simulink library "sm_rollerV_lib_underc_idlerArm_i2u0l3"  (R2026a)
settings: Solver=VariableStepAuto
undefined symbols (not defined in the file): Fixed, P1, P2, P3, P4, P5, Right, Trac, X, Y, Z
libraries: sm_rollerV_lib_underc_elem x11, sm_lib x11, nesl_utility x7, sm_trackV_lib_belt_underc_elem x4, fl_lib x2, sm_trackV_lib_frame_idlerArm_i2u0l3 x1
(part 1 of 2)
Description:
  | Copyright 2023-2026 The MathWorks, Inc.
settings Model: Creator=smiller  LastModifiedBy=smiller

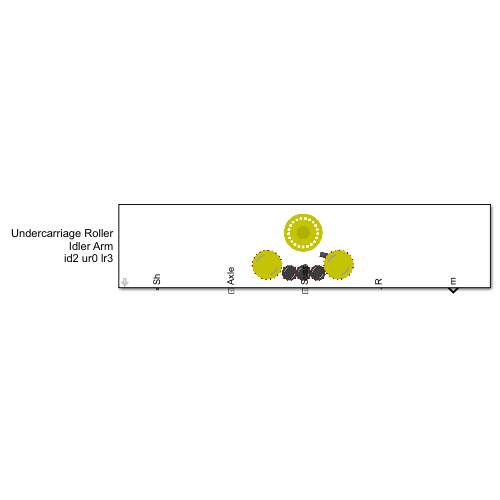
[thumbnail: Simulink's stored preview of the top-level diagram]
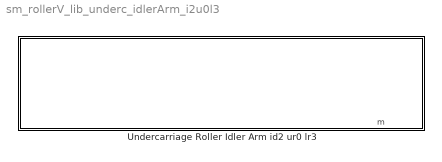
== system sm_rollerV_lib_underc_idlerArm_i2u0l3 ==
  Undercarriage Roller Idler Arm id2 ur0 lr3 : Subsystem  mask(Undercarriage with Roller Ground Contact (Point Cloud)){popup_leftOrRight=Right, sprk_rad_roll=Trac.Sprocket.Roller.rad, sprk_wid_roll=Trac.Sprocket.Roller.wid, sprk_clr=Trac.Sprocket.Roller.clr, sprk_opc=Trac.Sprocket.Roller.opc, sprk_rim_ir=Trac.Sprocket.Rim.rad_inner, sprk_rim_thk=Trac.Sprocket.Rim.thk, sprk_rim_spoke_xc=Trac.Sprocket.Rim.spoke_xc, sprk_rad_pitch=Trac.Sprocket.Spoke.pitch_rad, sprk_spoke_rad=Trac.Sprocket.Spoke.rad, sprk_spoke_len=Trac.Sprocket.Spoke.len, sprk_spoke_num=Trac.Sprocket.nSpokes, idlerR_rad=Trac.IdlerR.rad, idlerF_rad=Trac.IdlerF.rad, idlerR_total_len=Trac.IdlerR.len_total, idlerF_total_len=Trac.IdlerF.len_total, idlerR_avg_rho=Trac.IdlerR.rho_avg, idlerF_avg_rho=Trac.IdlerF.rho_avg, idlerR_clr=Trac.IdlerR.clr, idlerF_clr=Trac.IdlerF.clr, idlerR_opc=Trac.IdlerR.opc, idlerF_opc=Trac.IdlerF.opc, idlerR_contgeo_ptcld=Trac.IdlerR.ground_contact.ptcld.pts, idlerF_contgeo_ptcld=Trac.IdlerF.ground_contact.ptcld.pts, idlerR_contgeo_rad=Trac.IdlerR.ground_contact.ptcld.rad, idlerF_contgeo_rad=Trac.IdlerF.ground_contact.ptcld.rad, idlerR_contgeo_clr=Trac.IdlerR.belt_contact.clr, idlerF_contgeo_clr=Trac.IdlerF.belt_contact.clr, idlerR_contgeo_opc=Trac.IdlerR.belt_contact.opc, idlerF_contgeo_opc=Trac.IdlerF.belt_contact.opc, arm_idlerc=Trac.IdlerArm.Pivot_to_Idler, arm_tens_x=Trac.IdlerArm.Pivot_to_TensionerX, arm_tens_y=Trac.IdlerArm.Pivot_to_TensionerY, arm_wid=Trac.IdlerArm.wid, arm_thk=Trac.IdlerArm.thk, arm_rho=Trac.IdlerArm.rho, arm_clr=Trac.IdlerArm.clr, arm_opc=Trac.IdlerArm.opc, roller_lower_len=Trac.Roller.Lower.len, roller_lower_rad=Trac.Roller.Lower.rad, roller_lower_rho=Trac.Roller.Lower.rho, roller_lower_clr=Trac.Roller.Lower.clr, roller_lower_opc=Trac.Roller.Lower.opc, roller_lower_contgeo_clr=Trac.Roller.Lower.belt_contact.clr, roller_lower_contgeo_opc=Trac.Roller.Lower.belt_contact.opc, roller_lower_contgeo_ptcld=Trac.Roller.Lower.ground_contact.ptcld.pts, roller_lower_contgeo_rad=Trac.Roller.Lower.ground_contact.ptcld.rad, tensioner_cyl_len=Trac.IdlerF.Tensioner.cyl.len, tensioner_cyl_rad=Trac.IdlerF.Tensioner.cyl.rad, tensioner_cyl_rho=Trac.IdlerF.Tensioner.cyl.rho, tensioner_cyl_clr=Trac.IdlerF.Tensioner.cyl.clr, tensioner_cyl_opc=Trac.IdlerF.Tensioner.cyl.opc, tensioner_pist_len=Trac.IdlerF.Tensioner.piston.len, tensioner_pist_rad=Trac.IdlerF.Tensioner.piston.rad, tensioner_pist_rho=Trac.IdlerF.Tensioner.piston.rho, tensioner_pist_clr=Trac.IdlerF.Tensioner.piston.clr, tensioner_pist_opc=Trac.IdlerF.Tensioner.piston.opc, tensioner_br_len=Trac.IdlerF.Tensioner.bracket.len, tensioner_br_width=Trac.IdlerF.Tensioner.bracket.wid, tensioner_br_height=Trac.IdlerF.Tensioner.bracket.height, tensioner_br_thk=Trac.IdlerF.Tensioner.bracket.thk, tensioner_br_rho=Trac.IdlerF.Tensioner.bracket.rho, tensioner_br_clr=Trac.IdlerF.Tensioner.bracket.clr, tensioner_br_opc=Trac.IdlerF.Tensioner.bracket.opc, tensioner_eqpos=Trac.IdlerF.Tensioner.xeq, tensioner_x0=Trac.IdlerF.Tensioner.x0, tensioner_k=Trac.IdlerF.Tensioner.K, tensioner_b=Trac.IdlerF.Tensioner.B, popup_trackFrame=Fixed, roller_lower_x=Trac.Frame.SprkOffLon.Lower, axle_x=Trac.Frame.SprkOffLon.Axle, idlerFix_x=Trac.Frame.SprkOffLon.IdlerR, frame_pivot_x=Trac.Frame.SprkOffLon.PivotFra, tensionC_x=Trac.Frame.SprkOffLon.TensionC, idlerArm_x=Trac.Frame.SprkOffLon.IdlerArm, roller_lower_y=Trac.Frame.SprkOffVer.Lower, axle_y=Trac.Frame.SprkOffVer.Axle, idlerArm_y=Trac.Frame.SprkOffVer.IdlerArm, idlerFix_y=Trac.Frame.SprkOffVer.IdlerR, frame_pivot_y=Trac.Frame.SprkOffVer.PivotFra, tensionC_y=Trac.Frame.SprkOffVer.TensionC, frame_cg_offset=Trac.Frame.TrackFrame.CG, frame_mass=Trac.Frame.TrackFrame.Mass, frame_moi=Trac.Frame.TrackFrame.MOI, frame_poi=Trac.Frame.TrackFrame.POI, frame_roller_cg_offset=Trac.Frame.SprkFrame.CG, frame_roller_mass=Trac.Frame.SprkFrame.Mass, frame_roller_moi=Trac.Frame.SprkFrame.MOI, frame_roller_poi=Trac.Frame.SprkFrame.POI, frame_susp_offset=Trac.Frame.SuspOffset, roller_frame_pivot_range=Trac.Frame.PivotFra.Range, roller_frame_pivot_k=Trac.Frame.PivotFra.LimitK, roller_frame_pivot_b=Trac.Frame.PivotFra.LimitB, roller_frame_pivot_tw=Trac.Frame.PivotFra.LimitTW, sprk_rolling_rad=Trac.Sprocket.ground_contact.rolling_radius, roller_lower_rolling_rad=Trac.Roller.Lower.ground_contact.rolling_radius, idlerF_rolling_rad=Trac.IdlerF.ground_contact.rolling_radius, idlerR_rolling_rad=Trac.IdlerR.ground_contact.rolling_radius, rolling_cyl_len=Trac.Belt.w, accent_vis_lext=1e-3, roller_lower_cyl_clr=Trac.Roller.Lower.clr, roller_lower_cyl_opc=Trac.Roller.Lower.opc, idlerR_rollvervis_clr=Trac.IdlerR.clr, idlerF_rollvervis_clr=Trac.IdlerF.clr, idlerR_rollervis_opc=Trac.IdlerR.opc, idlerF_rollervis_opc=Trac.IdlerF.opc, accMn=0.65, accMx=0.75, acc_clr=[0.8 0.8 0.8], acc_opc=1, popup_sense_roller=Actuator Torque}
      mask prompts: popup_leftOrRight "Left or Right"; sprk_rad_roll "Rolling Radius (m)"; sprk_wid_roll "Roller Width (m)"; sprk_clr "Color [R G B] (0-1)"; sprk_opc "Roller Opacity (0-1)"; sprk_rim_ir "Inner Radius (m)"; sprk_rim_thk "Thickness (m)"; sprk_rim_spoke_xc "Spoke Cross Section [x y] (m)"; sprk_rad_pitch "Pitch Radius (m)"; sprk_spoke_rad "Radius (m)"; sprk_spoke_len "Length (m)"; sprk_spoke_num "Number of Spokes"; arm_idlerc "Offset Pivot to Idler Center (m)"; arm_tens_x "Offset Pivot to Tensioner Long. (m)"; arm_tens_y "Offset Pivot to Tensioner Vert. (m)"; arm_wid "Idler Arm Width (m)"; arm_thk "Idler Arm Thickness (m)"; arm_rho "Idler Arm Density"; arm_clr "Idler Arm Color [R G B] (m) (0-1)"; arm_opc "Opacity (0-1)"; roller_lower_len "Length (m)"; roller_lower_rad "Radius (m)"; roller_lower_rho "Density (kg/m^3)"; roller_lower_clr "Color [R G B] (0-1)"; roller_lower_opc "Opacity (0-1)"; roller_lower_contgeo_clr "Color [R G B] (0-1)"; roller_lower_contgeo_opc "Opacity (0-1)"; roller_lower_contgeo_ptcld "Point Cloud [x y z] (m)"; roller_lower_contgeo_rad "Radius (m)"; tensioner_cyl_len "Length (m)"; tensioner_cyl_rad "Radius (m)"; tensioner_cyl_rho "Density (kg/m^3)"; tensioner_cyl_clr "Color [R G B] (0-1)"; tensioner_cyl_opc "Opacity (0-1)"; tensioner_pist_len "Piston Length (m)"; tensioner_pist_rad "Radius (m)"; tensioner_pist_rho "Density (kg/m^3)"; tensioner_pist_clr "Color [R G B] (0-1)"; tensioner_pist_opc "Opacity (0.1)"; tensioner_br_len "Length (m)"; tensioner_br_width "Width (m)"; tensioner_br_height "Height (m)"; tensioner_br_thk "Bracket Thickness (m)"; tensioner_br_rho "Density (kg/m^3)"; tensioner_br_clr "Color [R G B] (0-1)"; tensioner_br_opc "Opacity (0.1)"; tensioner_eqpos "Equilibrium Position (m)"; tensioner_x0 "Assembly Position (m)"; tensioner_k "Stiffness Coefficient (N/m)"; tensioner_b "Damping Coefficient (N/(m/s))"; popup_trackFrame "Track Frame"; roller_lower_x "Lower Rollers (vector) (m)"; axle_x "Axle (m)"; idlerFix_x "Idler Wheel Fixed (m)"; frame_pivot_x "Frame Pivot (m)"; tensionC_x "Tensioner Cylinder (m)"; idlerArm_x "Idler Arm (m)"; roller_lower_y "Lower Rollers (m)"; axle_y "Axle (m)"; idlerArm_y "Idler Arm (m)"; idlerFix_y "Idler Wheel Fixed (m)"; frame_pivot_y "Frame Pivot (m)"; tensionC_y "Tensioner Cylinder (m)"; frame_cg_offset "CG Offset from Sprocket [x y z] (m)"; frame_mass "Mass (kg)"; frame_moi "Moments of Inertia [Ixx Iyy Izz] (kg*m^2)"; frame_poi "Products of Inertia [Ixx Iyy Izz] (kg*m^2)"; frame_roller_cg_offset "CG Offset from Sprocket [x y z] (m)"; frame_roller_mass "Mass (kg)"; frame_roller_moi "Moments of Inertia [Ixx Iyy Izz] (kg*m^2)"; frame_roller_poi "Products of Inertia [Ixx Iyy Izz] (kg*m^2)"; frame_susp_offset "Suspension Offset from Sprocket [x y z] (m)"; roller_frame_pivot_range "Range (deg)"; roller_frame_pivot_k "Stop stiffness (N*m/deg)"; roller_frame_pivot_b "Stop damping (N*m/(deg*sec)"; roller_frame_pivot_tw "Stop transition width (deg)"; sprk_rolling_rad "Sprocket Rolling Radius (m)"; roller_lower_rolling_rad "Lower Roller Rolling Radius (m)"; idlerF_rolling_rad "Front Idler Rolling Radius (m)"; idlerR_rolling_rad "Rear Idler Rolling Radius (m)"; rolling_cyl_len "Cylinder Length (m)"; accent_vis_lext "Length Extensions (m)"; roller_lower_cyl_clr "Cylinder Color [R G B] (0-1)"; roller_lower_cyl_opc "Cylinder Opacity (0-1)"; accMn "Accent Min Radius (0-1)"; accMx "Accent Max Radius (0-1)"; acc_clr "Accent Color [R G B] (0-1)"; acc_opc "Accent Opacity (0-1)"; popup_sense_roller "Roller"
      mask help: Models sprocket, rollers, fixed idler. and idler on an arm with a tensioner. Components have point cloud contact geometry to enable undercarriage to roll along uneven ground. The sprocket has a 1D rotational mechanical interface to the drivetrain.
      mask TypeOptions popup_leftOrRight: Frame/popup_leftOrRight
      mask TypeOptions sprk_rad_roll: Rollers/sprk_rad_roll
      mask TypeOptions sprk_wid_roll: Rollers/sprk_wid_roll
      mask TypeOptions sprk_clr: Rollers/sprk_clr
      mask TypeOptions sprk_opc: Rollers/sprk_opc
      mask TypeOptions sprk_rim_ir: Rollers/sprk_rim_ir
      mask TypeOptions sprk_rim_thk: Rollers/sprk_rim_thk
      mask TypeOptions sprk_rim_spoke_xc: Rollers/sprk_rim_spoke_xc
      mask TypeOptions sprk_rad_pitch: Rollers/sprk_rad_pitch
      mask TypeOptions sprk_spoke_rad: Rollers/sprk_spoke_rad
      mask TypeOptions sprk_spoke_len: Rollers/sprk_spoke_len
      mask TypeOptions sprk_spoke_num: Rollers/sprk_spoke_num
      mask TypeOptions idlerR_rad: Rollers/idlerR_rad
      mask TypeOptions idlerF_rad: Rollers/idlerF_rad
      mask TypeOptions idlerR_total_len: Rollers/idlerR_total_len
      mask TypeOptions idlerF_total_len: Rollers/idlerF_total_len
      mask TypeOptions idlerR_avg_rho: Rollers/idlerR_avg_rho
      mask TypeOptions idlerF_avg_rho: Rollers/idlerF_avg_rho
      mask TypeOptions idlerR_clr: Rollers/idlerR_clr
      mask TypeOptions idlerF_clr: Rollers/idlerF_clr
      mask TypeOptions idlerR_opc: Rollers/idlerR_opc
      mask TypeOptions idlerF_opc: Rollers/idlerF_opc
      mask TypeOptions idlerR_contgeo_ptcld: Rollers/idlerR_contgeo_ptcld
      mask TypeOptions idlerF_contgeo_ptcld: Rollers/idlerF_contgeo_ptcld
      mask TypeOptions idlerR_contgeo_rad: Rollers/idlerR_contgeo_rad
      mask TypeOptions idlerF_contgeo_rad: Rollers/idlerF_contgeo_rad
      mask TypeOptions idlerR_contgeo_clr: Rollers/idlerR_contgeo_clr
      mask TypeOptions idlerF_contgeo_clr: Rollers/idlerF_contgeo_clr
      mask TypeOptions idlerR_contgeo_opc: Rollers/idlerR_contgeo_opc
      mask TypeOptions idlerF_contgeo_opc: Rollers/idlerF_contgeo_opc
      mask TypeOptions arm_idlerc: Rollers/arm_idlerc
      mask TypeOptions arm_tens_x: Rollers/arm_tens_x
      mask TypeOptions arm_tens_y: Rollers/arm_tens_y
      mask TypeOptions arm_wid: Rollers/arm_wid
      mask TypeOptions arm_thk: Rollers/arm_thk
      mask TypeOptions arm_rho: Rollers/arm_rho
      mask TypeOptions arm_clr: Rollers/arm_clr
      mask TypeOptions arm_opc: Rollers/arm_opc
      mask TypeOptions roller_lower_len: Rollers/roller_lower_len
      mask TypeOptions roller_lower_rad: Rollers/roller_lower_rad
      mask TypeOptions roller_lower_rho: Rollers/roller_lower_rho
      mask TypeOptions roller_lower_clr: Rollers/roller_lower_clr
      mask TypeOptions roller_lower_opc: Rollers/roller_lower_opc
      mask TypeOptions roller_lower_contgeo_clr: Rollers/roller_lower_contgeo_clr
      mask TypeOptions roller_lower_contgeo_opc: Rollers/roller_lower_contgeo_opc
      mask TypeOptions roller_lower_contgeo_ptcld: Rollers/roller_lower_contgeo_ptcld
      mask TypeOptions roller_lower_contgeo_rad: Rollers/roller_lower_contgeo_rad
      mask TypeOptions tensioner_cyl_len: Rollers/tensioner_cyl_len
      mask TypeOptions tensioner_cyl_rad: Rollers/tensioner_cyl_rad
      mask TypeOptions tensioner_cyl_rho: Rollers/tensioner_cyl_rho
      mask TypeOptions tensioner_cyl_clr: Rollers/tensioner_cyl_clr
      mask TypeOptions tensioner_cyl_opc: Rollers/tensioner_cyl_opc
      mask TypeOptions tensioner_pist_len: Rollers/pist_len
      mask TypeOptions tensioner_pist_rad: Rollers/tensioner_pist_rad
      mask TypeOptions tensioner_pist_rho: Rollers/tensioner_pist_rho
      mask TypeOptions tensioner_pist_clr: Rollers/tensioner_pist_clr
      mask TypeOptions tensioner_pist_opc: Rollers/tensioner_pist_opc
      mask TypeOptions tensioner_br_len: Rollers/brk_len
      mask TypeOptions tensioner_br_width: Rollers/tensioner_br_width
      mask TypeOptions tensioner_br_height: Rollers/tensioner_br_height
      mask TypeOptions tensioner_br_thk: Rollers/brk_thk
      mask TypeOptions tensioner_br_rho: Rollers/tensioner_br_rho
      mask TypeOptions tensioner_br_clr: Rollers/tensioner_br_clr
      mask TypeOptions tensioner_br_opc: Rollers/tensioner_br_opc
      mask TypeOptions tensioner_eqpos: Rollers/tensioner_eqpos
      mask TypeOptions tensioner_x0: Rollers/tensioner_x0
      mask TypeOptions tensioner_k: Rollers/tensioner_k
      mask TypeOptions tensioner_b: Rollers/tensioner_b
      mask TypeOptions popup_trackFrame: Frame/popup_trackFrame
      mask TypeOptions roller_lower_x: Frame/roller_lower_x
      mask TypeOptions axle_x: Frame/axle_x
      mask TypeOptions idlerFix_x: Frame/idlerFix_x
      mask TypeOptions frame_pivot_x: Frame/frame_pivot_x
      mask TypeOptions tensionC_x: Frame/tensionC_x
      mask TypeOptions idlerArm_x: Frame/idlerArm_x
      mask TypeOptions roller_lower_y: Frame/roller_lower_y
      mask TypeOptions axle_y: Frame/axle_y
      mask TypeOptions idlerArm_y: Frame/idlerArm_y
      mask TypeOptions idlerFix_y: Frame/idlerFix_y
      mask TypeOptions frame_pivot_y: Frame/frame_pivot_y
      mask TypeOptions tensionC_y: Frame/tensionC_y
      mask TypeOptions frame_cg_offset: Frame/frame_cg_offset
      mask TypeOptions frame_mass: Frame/frame_mass
      mask TypeOptions frame_moi: Frame/frame_moi
      mask TypeOptions frame_poi: Frame/frame_poi
      mask TypeOptions frame_roller_cg_offset: Frame/frame_roller_cg_offset
      mask TypeOptions frame_roller_mass: Frame/frame_roller_mass
      mask TypeOptions frame_roller_moi: Frame/frame_roller_moi
      mask TypeOptions frame_roller_poi: Frame/frame_roller_poi
      mask TypeOptions frame_susp_offset: Frame/frame_susp_offset
      mask TypeOptions roller_frame_pivot_range: Frame/roller_frame_pivot_range
      mask TypeOptions roller_frame_pivot_k: Frame/roller_frame_pivot_k
      mask TypeOptions roller_frame_pivot_b: Frame/roller_frame_pivot_b
      mask TypeOptions roller_frame_pivot_tw: Frame/roller_frame_pivot_tw
      mask TypeOptions sprk_rolling_rad: Rollers/sprk_rolling_rad
      mask TypeOptions roller_lower_rolling_rad: Rollers/roller_lower_rolling_rad
      mask TypeOptions idlerF_rolling_rad: Rollers/idlerF_rolling_rad
      mask TypeOptions idlerR_rolling_rad: Rollers/idlerR_rolling_rad
      mask TypeOptions rolling_cyl_len: Rollers/cyl_len
      mask TypeOptions accent_vis_lext: Rollers/lext
      mask TypeOptions roller_lower_cyl_clr: Rollers/roller_lower_cyl_clr
      mask TypeOptions roller_lower_cyl_opc: Rollers/roller_lower_cyl_opc
      mask TypeOptions idlerR_rollvervis_clr: Rollers/idlerR_rollvervis_clr
      mask TypeOptions idlerF_rollvervis_clr: Rollers/idlerF_rollvervis_clr
      mask TypeOptions idlerR_rollervis_opc: Rollers/idlerR_rollervis_opc
      mask TypeOptions idlerF_rollervis_opc: Rollers/idlerF_rollervis_opc
      mask TypeOptions accMn: Rollers/accMn
      mask TypeOptions accMx: Rollers/accMx
      mask TypeOptions acc_clr: Rollers/acc_clr
      mask TypeOptions acc_opc: Rollers/acc_opc
      mask TypeOptions popup_sense_roller: Rollers/popup_sense_roller
      mask DialogControl cont_sprocket Prompt: Sprocket
      mask DialogControl cont_sprk_roller Prompt: Roller
      mask DialogControl cont_sprk_rim Prompt: Rim
      mask DialogControl cont_sprk_spoke Prompt: Spoke
      mask DialogControl cont_idler Prompt: Idler
      mask DialogControl cont_idler_roller Prompt: Roller
      mask DialogControl text_rear Prompt: Rear
      mask DialogControl text_front Prompt: Front
      mask DialogControl text_rad Prompt: Radius (m)
      mask DialogControl text_len Prompt: Total Length (m)
      mask DialogControl text_rho Prompt: Density (kg/m^3)
      mask DialogControl text_idler_clr Prompt: Color [R G B] (0-1)
      mask DialogControl text_idler_opc Prompt: Opacity (0-1)
      mask DialogControl cont_idler_contact_geo Prompt: Contact Geometry
      mask DialogControl text_idler_contgeo_ptcld Prompt: Point Cloud [x y z] (m)
      mask DialogControl text_idler_contgeo_rad Prompt: Radius (m)
      mask DialogControl text_contgeo_clr_copy Prompt: Color [R G B] (0-1)
      mask DialogControl text_contgeo_opc Prompt: Opacity (0-1)
      mask DialogControl cont_idler_arm Prompt: Idler Arm
      mask DialogControl cont_rollers Prompt: Rollers
      mask DialogControl cont_rollers_lower Prompt: Lower
      mask DialogControl cont_rollers_lower_contact_geo Prompt: Contact Geometry
      mask DialogControl cont_tensioner Prompt: Tensioner
      mask DialogControl cont_tensioner_cyl Prompt: Cylinder
      mask DialogControl cont_tensioner_pist Prompt: Piston
      mask DialogControl cont_tensioner_brkt Prompt: Bracket
      mask DialogControl cont_tensioner_assembly Prompt: Assembly
      mask DialogControl cont_frame Prompt: Frame
      mask DialogControl cont_offset_x Prompt: Longitudinal Offsets from Sprocket
      mask DialogControl cont_offset_y Prompt: Vertical Offsets
      mask DialogControl cont_mass Prompt: Mass and Inertia
      mask DialogControl cont_frame_sprk Prompt: Sprocket Frame
      mask DialogControl cont_frame_roller Prompt: Roller Frame
      mask DialogControl cont_susp Prompt: Suspension Offsets
      mask DialogControl cont_frame_pivot Prompt: Frame Pivot
      mask DialogControl cont_rolling Prompt: Rolling
      mask DialogControl cont_constraints_length Prompt: Constraints and Length
      mask DialogControl cont_rollervis_roller Prompt: Roller Visual: Roller
      mask DialogControl cont_rollervis_idler Prompt: Roller Visual: Idler
      mask DialogControl text_idler_rollervis_rear Prompt: Rear
      mask DialogControl text_idler_rollervis_front Prompt: Front
      mask DialogControl text_idler_rollervis_clr Prompt: Color [R G B] (0-1)
      mask DialogControl text_idler_rollervis_opc Prompt: Opacity (0-1)
      mask DialogControl cont_accentvis Prompt: Accent Visual
      mask DialogControl cont_sensing Prompt: Sensing
      mask Display: image('sm_roller_ptcld_rollers_idlerarm_i2u0l3_IMAGE.png')

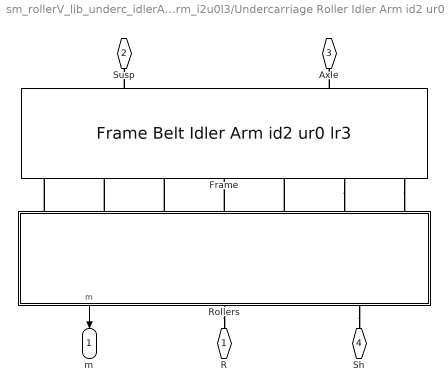
== system sm_rollerV_lib_underc_idlerArm_i2u0l3/Undercarriage Roller Idler Arm id2 ur0 lr3 ==
  Frame : sm_trackV_lib_frame_idlerArm_i2u0l3/Frame Belt Idler Arm id2 ur0 lr3  popup_leftOrRight=Right  popup_trackFrame=Fixed  roller_lower_x=roller_lower_x  idlerArm_x=idlerArm_x  idlerFix_x=idlerFix_x  tensionC_x=tensionC_x  frame_pivot_x=frame_pivot_x  axle_x=axle_x  roller_lower_y=roller_lower_y  idlerArm_y=idlerArm_y  idlerFix_y=idlerFix_y  tensionC_y=tensionC_y  frame_pivot_y=frame_pivot_y  axle_y=axle_y  frame_roller_cg_offset=frame_roller_cg_offset  frame_roller_mass=frame_roller_mass  frame_roller_moi=frame_roller_moi  frame_roller_poi=frame_roller_poi  frame_cg_offset=frame_cg_offset  frame_mass=frame_mass  frame_moi=frame_moi  frame_poi=frame_poi  frame_susp_offset=frame_susp_offset  roller_frame_pivot_range=roller_frame_pivot_range  roller_frame_pivot_k=roller_frame_pivot_k  roller_frame_pivot_b=roller_frame_pivot_b  roller_frame_pivot_tw=roller_frame_pivot_tw
  Rollers : Subsystem  mask(Rollers for Integration with Track Model){sprk_wid_roll=sprk_wid_roll, sprk_rad_roll=sprk_rad_roll, sprk_clr=sprk_clr, sprk_opc=sprk_opc, sprk_rim_ir=sprk_rim_ir, sprk_rim_spoke_xc=sprk_rim_spoke_xc, sprk_rim_thk=sprk_rim_thk, sprk_rad_pitch=sprk_rad_pitch, sprk_spoke_rad=sprk_spoke_rad, sprk_spoke_len=sprk_spoke_len, sprk_spoke_num=sprk_spoke_num, idlerR_rad=idlerR_rad, idlerF_rad=idlerF_rad, idlerR_total_len=idlerR_total_len, idlerF_total_len=idlerF_total_len, idlerR_avg_rho=idlerR_avg_rho, idlerF_avg_rho=idlerF_avg_rho, idlerR_clr=idlerR_clr, idlerF_clr=idlerF_clr, idlerR_opc=idlerR_opc, idlerF_opc=idlerF_opc, idlerR_contgeo_ptcld=idlerR_contgeo_ptcld, idlerF_contgeo_ptcld=idlerF_contgeo_ptcld, idlerR_contgeo_rad=idlerR_contgeo_rad, idlerF_contgeo_rad=idlerF_contgeo_rad, idlerR_contgeo_clr=idlerR_contgeo_clr, idlerF_contgeo_clr=idlerF_contgeo_clr, idlerR_contgeo_opc=idlerR_contgeo_opc, idlerF_contgeo_opc=idlerF_contgeo_opc, arm_idlerc=arm_idlerc, arm_tens_x=arm_tens_x, arm_tens_y=arm_tens_y, arm_wid=arm_wid, arm_thk=arm_thk, arm_rho=arm_rho, arm_clr=arm_clr, arm_opc=arm_opc, roller_lower_len=roller_lower_len, roller_lower_rad=roller_lower_rad, roller_lower_rho=roller_lower_rho, roller_lower_clr=roller_lower_clr, roller_lower_opc=roller_lower_opc, roller_lower_contgeo_ptcld=roller_lower_contgeo_ptcld, roller_lower_contgeo_rad=roller_lower_contgeo_rad, roller_lower_contgeo_clr=roller_lower_contgeo_clr, roller_lower_contgeo_opc=roller_lower_contgeo_opc, tensioner_cyl_rad=tensioner_cyl_rad, tensioner_cyl_len=tensioner_cyl_len, tensioner_cyl_rho=tensioner_cyl_rho, tensioner_cyl_clr=tensioner_cyl_clr, tensioner_cyl_opc=tensioner_cyl_opc, tensioner_pist_rad=tensioner_pist_rad, pist_len=tensioner_pist_len, tensioner_pist_rho=tensioner_pist_rho, tensioner_pist_clr=tensioner_pist_clr, tensioner_pist_opc=tensioner_pist_opc, brk_len=tensioner_br_len, tensioner_br_width=tensioner_br_width, tensioner_br_height=tensioner_br_height, brk_thk=tensioner_br_thk, tensioner_br_rho=tensioner_br_rho, tensioner_br_clr=tensioner_br_clr, tensioner_br_opc=tensioner_br_opc, tensioner_eqpos=tensioner_eqpos, tensioner_x0=tensioner_x0, tensioner_b=tensioner_b, tensioner_k=tensioner_k, sprk_rolling_rad=sprk_rolling_rad, roller_lower_rolling_rad=roller_lower_rolling_rad, idlerF_rolling_rad=idlerF_rolling_rad, idlerR_rolling_rad=idlerR_rolling_rad, cyl_len=rolling_cyl_len, roller_lower_cyl_clr=roller_lower_cyl_clr, roller_lower_cyl_opc=roller_lower_cyl_opc, idlerR_rollvervis_clr=idlerR_rollvervis_clr, idlerF_rollvervis_clr=idlerF_rollvervis_clr, idlerR_rollervis_opc=idlerR_rollervis_opc, idlerF_rollervis_opc=idlerF_rollervis_opc, accMn=accMn, accMx=accMx, acc_clr=acc_clr, acc_opc=acc_opc, lext=accent_vis_lext, popup_sense_roller=Actuator Torque}
      mask prompts: sprk_wid_roll "Roller Width (m)"; sprk_rad_roll "Rolling Radius (m)"; sprk_clr "Roller Color [R G B] (0-1)"; sprk_opc "Roller Opacity (0-1)"; sprk_rim_ir "Inner Radius (m)"; sprk_rim_spoke_xc "Spoke Cross Section [x y] (m)"; sprk_rim_thk "Thickness (m)"; sprk_rad_pitch "Pitch Radius (m)"; sprk_spoke_rad "Radius (m)"; sprk_spoke_len "Length (m)"; sprk_spoke_num "Number of Spokes"; arm_idlerc "Offset Pivot to Idler Center (m)"; arm_tens_x "Offset Pivot to Tensioner Long.  (m)"; arm_tens_y "Offset Pivot to Tensioner Vert.  (m)"; arm_wid "Idler Arm Width (m)"; arm_thk "Idler Arm Thickness (m)"; arm_rho "Idler Arm Density (kg/m^3)"; arm_clr "Idler Arm Color [R G B] (0-1)"; arm_opc "Idler Arm Opacity (0-1)"; roller_lower_len "Length (m)"; roller_lower_rad "Radius (m)"; roller_lower_rho "Density (kg/m^3)"; roller_lower_clr "Color [R G B] (0-1)"; roller_lower_opc "Opacity (0-1)"; roller_lower_contgeo_ptcld "Point Cloud [x y z] (m)"; roller_lower_contgeo_rad "Radius (m)"; roller_lower_contgeo_clr "Color [R G B] (0-1)"; roller_lower_contgeo_opc "Opacity (0-1)"; tensioner_cyl_rad "Radius (m)"; tensioner_cyl_len "Length (m)"; tensioner_cyl_rho "Density (kg/m^3)"; tensioner_cyl_clr "Color [R G B] (0-1)"; tensioner_cyl_opc "Opacity (0-1)"; tensioner_pist_rad "Radius (m)"; pist_len "Piston Length (m)"; tensioner_pist_rho "Density (kg/m^3)"; tensioner_pist_clr "Color [R G B] (0-1)"; tensioner_pist_opc "Opacity (0.1)"; brk_len "Bracket Length (m)"; tensioner_br_width "Width (m)"; tensioner_br_height "Height (m)"; brk_thk "Bracket Thickness (m)"; tensioner_br_rho "Density (kg/m^3)"; tensioner_br_clr "Color [R G B] (0-1)"; tensioner_br_opc "Opacity (0.1)"; tensioner_eqpos "Equilibrium Position (m)"; tensioner_x0 "Assembly Position (m)"; tensioner_b "Damping Coefficient (N/(m/s))"; tensioner_k "Stiffness Coefficient (N/m)"; sprk_rolling_rad "Sprocket Rolling Radius (m)"; roller_lower_rolling_rad "Lower Roller Rolling Radius (m)"; idlerF_rolling_rad "Front Idler Rolling Radius (m)"; idlerR_rolling_rad "Rear Idler Rolling Radius (m)"; cyl_len "Cylinder Length (m)"; roller_lower_cyl_clr "Cylinder Color [R G B] (0-1)"; roller_lower_cyl_opc "Cylinder Opacity (0-1)"; accMn "Accent Min Radius (0-1)"; accMx "Accent Max Radius (0-1)"; acc_clr "Accent Color [R G B] (0-1)"; acc_opc "Accent Opacity (0-1)"; lext "Length Extensions (m)"; popup_sense_roller "Roller"
      mask help: Models sprocket, rollers, and idler with tensioner. Components have contact geometry for integration with a segmented track model. The sprocket has a 1D rotational mechanical interface to the drivetrain.
      mask init:
      | % Sensing a constraint force can be computationally expensive
      | % Use popup to turn it off if quantity is not needed
      | 
      | bh = gcb;
      | if(strcmp(get_param(bh,'popup_sense_roller'),'Constraint Force'))
      |     SCF = 'on'; STF = 'off';
      |     connectedPort = "fc_out";
      |     senseConstraintTorque = "on";
      |     senseTorqueForce = "off";
      | 
      | else
      |     SCF = 'off'; STF = 'on';
      |     connectedPort = "t_out";
      |     senseConstraintTorque = "off";
      |     senseTorqueForce = "on";
      | end
      | 
      | f = Simulink.FindOptions('RegExp',true,'SearchDepth',1);
      | bh_rv = Simulink.findBlocks(gcb,'Name','Revolute Lower #*',f);
      | bh_ps = Simulink.findBlocks(bh,'Name','PS-SL Lower #*',f);
      | [~, indrv] = sort(getfullname(bh_rv));
      | [~, indps] = sort(getfullname(bh_ps));
      | bh_rv = bh_rv(indrv);
      | bh_ps = bh_ps(indps);
      | 
      | bh_rvidf = get_param([bh '/Revolute Idler F'],'Handle');
      | bh_rvidr = get_param([bh '/Revolute Idler R'],'Handle');
      | 
      | bh_psidf = get_param([bh '/PS-SL IdlerF'],'Handle');
      | bh_psidr = get_param([bh '/PS-SL IdlerR'],'Handle');
      | 
      | bh_rv = [bh_rv; bh_rvidr; bh_rvidf];
      | bh_ps = [bh_ps; bh_psidr; bh_psidf];
      | 
      | for i = 1:length(bh_rv)
      |     port_rv = get_param(bh_rv(i),'PortHandles');
      |     port_ps = get_param(bh_ps(i),'PortHandles');
      |     line_rv = get_param(bh_rv(i),'LineHandles');
      |     delete_line(line_rv.RConn(2))
      |     set_param(bh_rv(i),'SenseConstraintForce',SCF,'SenseTorqueForce',STF);
      |     simscape.addConnection(bh_rv(i), connectedPort, bh_ps(i),'input');
      | end
      mask TypeOptions sprk_wid_roll: Sprocket/sprk_wid_roll
      mask TypeOptions sprk_rad_roll: Sprocket/sprk_rad_roll
      mask TypeOptions sprk_clr: Sprocket/sprk_clr | Sprocket/sprk_spoke_clr
      mask TypeOptions sprk_opc: Sprocket/sprk_opc | Sprocket/sprk_spoke_opc
      mask TypeOptions sprk_rim_ir: Sprocket/rim_ir
      mask TypeOptions sprk_rim_spoke_xc: Sprocket/rim_spoke_xc
      mask TypeOptions sprk_rim_thk: Sprocket/rim_thk
      mask TypeOptions sprk_rad_pitch: Sprocket/sprk_rad_pitch
      mask TypeOptions sprk_spoke_rad: Sprocket/sprk_spoke_rad
      mask TypeOptions sprk_spoke_len: Sprocket/sprk_spoke_len
      mask TypeOptions sprk_spoke_num: Sprocket/sprk_spoke_num
      mask TypeOptions idlerR_rad: IdlerR/roller_lower_rad
      mask TypeOptions idlerF_rad: IdlerF/roller_lower_rad
      mask TypeOptions idlerR_total_len: IdlerR/roller_lower_len
      mask TypeOptions idlerF_total_len: IdlerF/roller_lower_len
      mask TypeOptions idlerR_avg_rho: IdlerR/roller_lower_rho
      mask TypeOptions idlerF_avg_rho: IdlerF/roller_lower_rho
      mask TypeOptions idlerR_clr: IdlerR/roller_lower_clr
      mask TypeOptions idlerF_clr: IdlerF/roller_lower_clr
      mask TypeOptions idlerR_opc: IdlerR/roller_lower_opc
      mask TypeOptions idlerF_opc: IdlerF/roller_lower_opc
      mask TypeOptions idlerR_contgeo_ptcld: IdlerR/roller_lower_contgeo_ptcld
      mask TypeOptions idlerF_contgeo_ptcld: IdlerF/roller_lower_contgeo_ptcld
      mask TypeOptions idlerR_contgeo_rad: IdlerR/roller_lower_contgeo_rad
      mask TypeOptions idlerF_contgeo_rad: IdlerF/roller_lower_contgeo_rad
      mask TypeOptions idlerR_contgeo_clr: IdlerR/roller_lower_contgeo_clr
      mask TypeOptions idlerF_contgeo_clr: IdlerF/roller_lower_contgeo_clr
      mask TypeOptions idlerR_contgeo_opc: IdlerR/roller_lower_contgeo_opc
      mask TypeOptions idlerF_contgeo_opc: IdlerF/roller_lower_contgeo_opc
      mask TypeOptions arm_idlerc: Arm/arm_idlerc
      mask TypeOptions arm_tens_x: Arm/arm_tens_x
      mask TypeOptions arm_tens_y: Arm/arm_tens_y
      mask TypeOptions arm_wid: Arm/arm_wid
      mask TypeOptions arm_thk: Arm/arm_thk
      mask TypeOptions arm_rho: Arm/arm_rho
      mask TypeOptions arm_clr: Arm/arm_clr
      mask TypeOptions arm_opc: Arm/arm_opc
      mask TypeOptions roller_lower_len:
      | Roller
      | Lower 1/roller_lower_len | Roller
      | Lower 2/roller_lower_len | Roller
      | Lower 3/roller_lower_len
      mask TypeOptions roller_lower_rad:
      | Roller
      | Lower 1/roller_lower_rad | Roller
      | Lower 2/roller_lower_rad | Roller
      | Lower 3/roller_lower_rad
      mask TypeOptions roller_lower_rho:
      | Roller
      | Lower 1/roller_lower_rho | Roller
      | Lower 2/roller_lower_rho | Roller
      | Lower 3/roller_lower_rho
      mask TypeOptions roller_lower_clr:
      | Roller
      | Lower 1/roller_lower_clr | Roller
      | Lower 2/roller_lower_clr | Roller
      | Lower 3/roller_lower_clr
      mask TypeOptions roller_lower_opc:
      | Roller
      | Lower 1/roller_lower_opc | Roller
      | Lower 2/roller_lower_opc | Roller
      | Lower 3/roller_lower_opc
      mask TypeOptions roller_lower_contgeo_ptcld:
      | Roller
      | Lower 1/roller_lower_contgeo_ptcld | Roller
      | Lower 2/roller_lower_contgeo_ptcld | Roller
      | Lower 3/roller_lower_contgeo_ptcld
      mask TypeOptions roller_lower_contgeo_rad:
      | Roller
      | Lower 1/roller_lower_contgeo_rad | Roller
      | Lower 2/roller_lower_contgeo_rad | Roller
      | Lower 3/roller_lower_contgeo_rad
      mask TypeOptions roller_lower_contgeo_clr:
      | Roller
      | Lower 1/roller_lower_contgeo_clr | Roller
      | Lower 2/roller_lower_contgeo_clr | Roller
      | Lower 3/roller_lower_contgeo_clr | Roller
      | Lower 4/roller_lower_contgeo_clr
      mask TypeOptions roller_lower_contgeo_opc:
      | Roller
      | Lower 1/roller_lower_contgeo_opc | Roller
      | Lower 2/roller_lower_contgeo_opc | Roller
      | Lower 3/roller_lower_contgeo_opc | Roller
      | Lower 4/roller_lower_contgeo_opc
      mask TypeOptions tensioner_cyl_rad:
      | Tensioner
      | Cylinder/cyl_rad
      mask TypeOptions tensioner_cyl_len:
      | Tensioner
      | Cylinder/cyl_len
      mask TypeOptions tensioner_cyl_rho:
      | Tensioner
      | Cylinder/cyl_rho
      mask TypeOptions tensioner_cyl_clr:
      | Tensioner
      | Cylinder/cyl_clr
      mask TypeOptions tensioner_cyl_opc:
      | Tensioner
      | Cylinder/cyl_opc
      mask TypeOptions tensioner_pist_rad:
      | Tensioner
      | Piston/pist_rad
      mask TypeOptions pist_len:
      | Tensioner
      | Cylinder/pist_len | Tensioner
      | Piston/pist_len
      mask TypeOptions tensioner_pist_rho:
      | Tensioner
      | Piston/pist_rho
      mask TypeOptions tensioner_pist_clr:
      | Tensioner
      | Piston/pist_clr
      mask TypeOptions tensioner_pist_opc:
      | Tensioner
      | Piston/pist_opc
      mask TypeOptions brk_len:
      | Tensioner
      | Cylinder/brk_len | Tensioner
      | Piston/br_length
      mask TypeOptions tensioner_br_width:
      | Tensioner
      | Piston/br_width
      mask TypeOptions tensioner_br_height:
      | Tensioner
      | Piston/br_height
      mask TypeOptions brk_thk:
      | Tensioner
      | Cylinder/brk_thk | Tensioner
      | Piston/br_thk
      mask TypeOptions tensioner_br_rho:
      | Tensioner
      | Piston/br_rho
      mask TypeOptions tensioner_br_clr:
      | Tensioner
      | Piston/br_clr
      mask TypeOptions tensioner_br_opc:
      | Tensioner
      | Piston/br_opc
      mask TypeOptions tensioner_eqpos:
      | Prismatic
      | Tensioner/EquilibriumPosition
      mask TypeOptions tensioner_x0:
      | Prismatic
      | Tensioner/PositionTargetValue
      mask TypeOptions tensioner_b:
      | Prismatic
      | Tensioner/DampingCoefficient
      mask TypeOptions tensioner_k:
      | Prismatic
      | Tensioner/SpringStiffness
      mask TypeOptions sprk_rolling_rad:
      | Constrain
      | Rollers
      | Idlers/sprk_rolling_rad
      mask TypeOptions roller_lower_rolling_rad:
      | Constrain
      | Rollers
      | Idlers/roller_lower_rolling_rad | Roller
      | Lower 1/cyl_rad | Roller
      | Lower 2/cyl_rad | Roller
      | Lower 3/cyl_rad
      mask TypeOptions idlerF_rolling_rad:
      | Constrain
      | Rollers
      | Idlers/idlerF_rolling_rad | IdlerF/cyl_rad
      mask TypeOptions idlerR_rolling_rad:
      | Constrain
      | Rollers
      | Idlers/idlerR_rolling_rad | IdlerR/cyl_rad
      mask TypeOptions cyl_len:
      | IdlerF/cyl_len | IdlerR/cyl_len | Roller
      | Lower 1/cyl_len | Roller
      | Lower 2/cyl_len | Roller
      | Lower 3/cyl_len
      mask TypeOptions roller_lower_cyl_clr:
      | Roller
      | Lower 1/cyl_clr | Roller
      | Lower 2/cyl_clr | Roller
      | Lower 3/cyl_clr
      mask TypeOptions roller_lower_cyl_opc:
      | Roller
      | Lower 1/cyl_opc | Roller
      | Lower 2/cyl_opc | Roller
      | Lower 3/cyl_opc
      mask TypeOptions idlerR_rollvervis_clr: IdlerR/cyl_clr
      mask TypeOptions idlerF_rollvervis_clr: IdlerF/cyl_clr
      mask TypeOptions idlerR_rollervis_opc: IdlerR/cyl_opc
      mask TypeOptions idlerF_rollervis_opc: IdlerF/cyl_opc
      mask TypeOptions accMn:
      | IdlerF/accMn | IdlerR/accMn | Roller
      | Lower 1/accMn | Roller
      | Lower 2/accMn | Roller
      | Lower 3/accMn
      mask TypeOptions accMx:
      | IdlerF/accMx | IdlerR/accMx | Roller
      | Lower 1/accMx | Roller
      | Lower 2/accMx | Roller
      | Lower 3/accMx
      mask TypeOptions acc_clr:
      | IdlerF/acc_clr | IdlerR/acc_clr | Roller
      | Lower 1/acc_clr | Roller
      | Lower 2/acc_clr | Roller
      | Lower 3/acc_clr
      mask TypeOptions acc_opc:
      | IdlerF/acc_opc | IdlerR/acc_opc | Roller
      | Lower 1/acc_opc | Roller
      | Lower 2/acc_opc | Roller
      | Lower 3/acc_opc
      mask TypeOptions lext:
      | IdlerF/lext | IdlerR/lext | Roller
      | Lower 1/lext | Roller
      | Lower 2/lext | Roller
      | Lower 3/lext
      mask TypeOptions popup_sense_roller: Constraint Force | Actuator Torque
      mask DialogControl cont_sprk Prompt: Sprocket
      mask DialogControl sprk_roller Prompt: Roller
      mask DialogControl cont_rim Prompt: Rim
      mask DialogControl sprk_spoke Prompt: Spoke
      mask DialogControl cont_idler Prompt: Idler
      mask DialogControl cont_idler_roller Prompt: Roller
      mask DialogControl text_idler_rear Prompt: Rear
      mask DialogControl text_idler_front Prompt: Front
      mask DialogControl text_radius Prompt: Radius (m)
      mask DialogControl text_len Prompt: Total Length(m)
      mask DialogControl text_rho Prompt: Average Density (kg/m^3)
      mask DialogControl text_idler_clr Prompt: Color [R G B] (0-1)
      mask DialogControl text_idler_opc Prompt: Opacity (0-1)
      mask DialogControl cont_idler_contact_geo Prompt: Contact Geometry
      mask DialogControl text_idler_contgeo_ptcld Prompt: Point Cloud [x y z] (m)
      mask DialogControl text_idler_contgeo_rad Prompt: Radius (m)
      mask DialogControl text_idler_contgeo_clr Prompt: Color [R G B] (0-1)
      mask DialogControl text_idler_contgeo_opc Prompt: Opacity (0-1)
      mask DialogControl cont_idlerArm Prompt: Idler Arm
      mask DialogControl cont_rollers Prompt: Rollers
      mask DialogControl cont_lower Prompt: Lower
      mask DialogControl cont_lower_contact_geo Prompt: Contact Geometry
      mask DialogControl cont_tensioner Prompt: Tensioner
      mask DialogControl cont_tensioner_cyl Prompt: Cylinder
      mask DialogControl cont_tensioner_pist Prompt: Piston
      mask DialogControl cont_tensioner_brkt Prompt: Bracket
      mask DialogControl cont_tensioner_assy Prompt: Assembly
      mask DialogControl cont_rolling Prompt: Rolling
      mask DialogControl cont_constr_and_length Prompt: Constraints and Length
      mask DialogControl cont_lower_rollervis Prompt: Roller Visual: Roller
      mask DialogControl cont_idler_rollervis Prompt: Roller Visual: Idler
      mask DialogControl text_idler_rollervis_clr Prompt: Cylinder Color (m)
      mask DialogControl text_idler_rollervis_opc Prompt: Cylinder Opacity (0-1)
      mask DialogControl Container25 Prompt: Accent Visual
      mask DialogControl Container20 Prompt: Sensing
      mask Display: image('sm_roller_ptcld_rollers_idlerarm_i2u0l3_IMAGE.png');
  R : PMIOPort  Side=Right
  Susp : PMIOPort  Port=2  Side=Right
  Axle : PMIOPort  Port=3  Side=Right
  Sh : PMIOPort  Port=4  Side=Right
  m : Outport
  wires:
  Rollers/1(m) -> m/1
  connections:
  Rollers/LConn1 -- Frame/RConn1
  Rollers/RConn2 -- Sh/RConn1
  Frame/LConn2 -- Axle/RConn1
  Rollers/RConn1 -- R/RConn1
  Frame/LConn1 -- Susp/RConn1
  Frame/RConn6 -- Rollers/LConn6
  Rollers/LConn5 -- Frame/RConn5
  Rollers/LConn4 -- Frame/RConn4
  Rollers/LConn3 -- Frame/RConn3
  Rollers/LConn2 -- Frame/RConn2
  Frame/RConn7 -- Rollers/LConn7
